simulink model "segway_2015"  (R2015a)
settings: Solver=ode45  StartTime=0.0  StopTime=5  RelTol=1e-6  AbsTol=1e-9
values from neighbouring files (symbols this model uses):
  param = [M m Ith Imr h W R Ke Rm Trmax Dm n]    [CONTROL_SEGWAY.m]    (also in Control_Segway_2015.m; ensayo1.mat = [0.6 0.034 0.001425 0.0037532 0.073 0.15 0.0408 0.01 4.5 0 0; ensayo2_wn4.8_seta_0.7.mat = [0.6 0.034 0.001425 0.0037532 0.073 0.15 0.0408 0.01 4.5 0 0; ensayo3_wn5.3_seta_0.55.mat = [0.6 0.034 0.001425 0.0037532 0.073 0.15 0.0408 0.01 4.5 0 0)
settings Model: CovHtmlReporting=off  CovSFcnEnable=off  Creator=zamora  LastModifiedBy=stic
settings DataIOCC: SignalLoggingSaveFormat=ModelDataLogs
settings OptimizationCC: ExpressionDepthLimit=2147483647
settings DebuggingCC: UnderspecifiedInitializationDetection=Classic  MergeDetectMultiDrivingBlocksExec=none  MultiTaskDSMMsg=warning  MultiTaskCondExecSysMsg=none  FcnCallInpInsideContextMsg=EnableAllAsWarning  StateNameClashWarn=warning
settings GRTTargetCC: CombineOutputUpdateFcns=off  GRTInterface=on

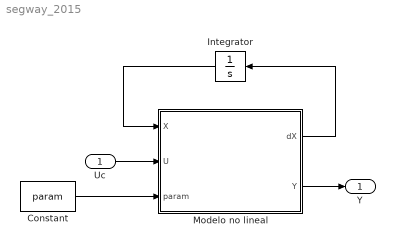
== system segway_2015 ==
  Uc : Inport
  Constant : Constant  Value=param  SampleTime=0
  Integrator : Integrator  InitialCondition=zeros(3,1)
  Modelo no lineal : MATLAB Function  TreatAsAtomicUnit=on
      settings: PermitHierarchicalResolution=ParametersOnly
  Y : Outport
  wires:
  Modelo no lineal/1(dX) -> Integrator/1
  Integrator/1 -> Modelo no lineal/1(X)
  Constant/1 -> Modelo no lineal/3(param)
  Modelo no lineal/2(Y) -> Y/1
  Uc/1 -> Modelo no lineal/2(U)

== matlab function segway_2015/Modelo no lineal ==
  data: X input; dX output; U input; param input; Y output
function [dX,Y] = segway(X,U,param)

%% Parametros
% Masa del chasis (kg)
M=param(1);
% Masa de la rueda incluyendo el rotor del motor (kg)
m=param(2);
% Momento de inercia de cabeceo del chasis (kg.m^2)
Ith=param(3);
% Momento de inercia del conjunto motor + rueda (kg.m^2)
Imr=param(4);
% Distancia al centro de gravedad del chasis medida desde el eje (m)
h=param(5);
% Distancia de separacion entre ruedas (m)
W=param(6);
% Radio de las rueda (m)
R=param(7);
% Constante electrica del motor (V.s/rad)
Ke=param(8);
% Constante mecanica del motor (N.m/A)
Kt=Ke;
% Resistencia electrica del motor
Rm=param(9);
% Par de friccion del motor (N.m) eje externo
Trmax=param(10);
% Coeficiente de friccion viscosa eje externo (N.m.s/rad)
Dm=param(11);
% Relacion de engranajes
n=param(12);


% Gravedad (m/s^2)
g=9.81;

%% Entradas
% Tension comun (V)
uc=U(1);

%% Variables de estado
% Velocidad comun lineal de las ruedas (m/s)
vRc=X(1);
% Velocidad angular de cabeceo (rad/s)
wth=X(2);
% Angulo de cabeceo (rad)
th=X(3);
% Velocidad angular de la rueda (rad/s)
wRc=vRc/R;
% Velocidad angular del motor
wmc=n*wRc-wth;


%% Motor
% Ecuacion electrica del motor
ic=(uc-Ke*wmc)/Rm;
% Par motor eje motor
Tmc=Kt*ic;
% Par motor límite (eje motor) para aplicación del par máximo de fricción (eje rueda)
wmc_aux = 5*[-2 -1 1 2];
Trc_aux = Trmax/n*[-1 -1 1 1];
% Tmc_lim=Tmc*(Tmc>-Trmax/n && Tmc<Trmax/n)-Trmax/n*(Tmc<=-Trmax/n)+Trmax*(Tmc>=Trmax/n);
% Par de friccion estatico (eje rueda)
% Trc=n*Tmc_lim*(abs(wmc)==0)+Trmax*sign(wmc)*(abs(wmc)>0);
Trc = interp1(wmc_aux,Trc_aux,wmc,'linear','extrap');
% Par neto (eje motor)
Tc=Tmc-Dm*wRc/n-Trc/n;

%% Avance del vehiculo y cabeceo
% 2*n*Tc/R = (2*(m+Imr/R^2)+M)*aRc + M*h*alfath*cos(th) - M*wth^2*h*sin(th)
% -2*Tc + M*g*h*sin(th) = M*h*cos(th)*aRc + (Ith+M*h^2)*alfath
% Se resuelve el sistema de ecuaciones anterior
matA_aux=[2*(m+Imr/R^2)+M   M*h*cos(th)
              M*h*cos(th)   Ith+M*h^2];
matB_aux=[2*n*Tc/R + M*wth^2*h*sin(th) ; -2*Tc + M*g*h*sin(th)];
aux=matA_aux\matB_aux;
aRc=aux(1);
alfath=aux(2); 

% Derivada del vector de estado
dX=[aRc alfath wth]';

%% Ecuaciones de salida
Y = X;
